simulink model "gm_sampleModel1449_sub"  (R2023a)
settings: Solver=VariableStepAuto  StartTime=0.0  StopTime=10.0  RelTol=1e-3
libraries: hdlsllib x1, simulink x1
settings Model: Creator=user1  LastModifiedBy=user1
settings OptimizationCC: BlockReduction=off  ConditionallyExecuteInputs=off
settings DebuggingCC: InheritedTsInSrcMsg=none

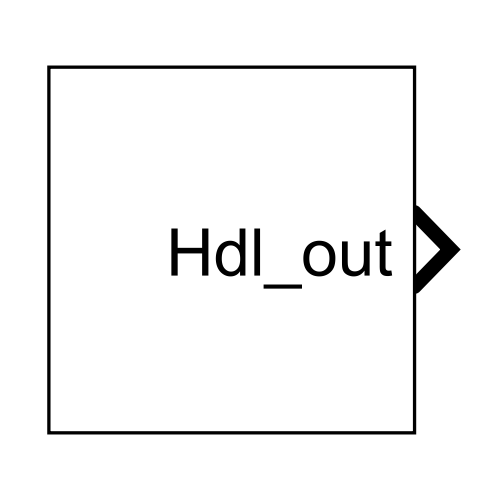
[thumbnail: Simulink's stored preview of the top-level diagram]
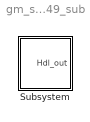
== system gm_sampleModel1449_sub ==
  Subsystem : Subsystem

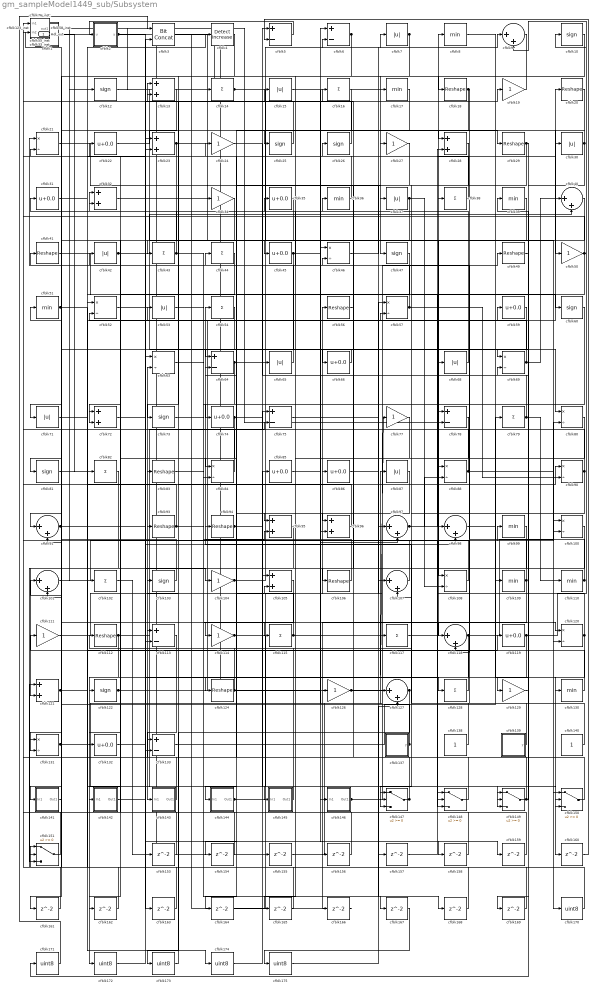
== system gm_sampleModel1449_sub/Subsystem ==
  cfblk1 : Subsystem  mask(Detect Rise Positive){vinit=double(0), InputProcessing=Elements as channels (sample based), OutDataTypeStr=uint8}
      mask prompts: vinit "Simulink:masks:InitialCondition_MP"; InputProcessing "Simulink:masks:InputProcessing_MP"; OutDataTypeStr "Simulink:masks:OutputDataType_MP"
      mask help: Simulink:masks:DetectRisePositive_MD
      mask init:
      | InputProcessing = 'Elements as channels (sample based)';
      | OutDataTypeStr = 'uint8';
      | vinit = double(0);
      mask TypeOptions InputProcessing: Simulink:masks:ColumnsAsChannelsFrameBased | Simulink:masks:ElementsAsChannelsSampleBased
      mask TypeOptions OutDataTypeStr: Simulink:masks:uint8 | Simulink:masks:boolean
      mask Display: fprintf('U > 0\n&  NOT\nU/z > 0')
  cfblk{10,12,25..26,47,60,73,81,103,122} (10 alike) : Signum
  cfblk{21,46,52,57,63,69,80,84,88,90,100,108,120,131} (14 alike) : Product  Inputs=*/  OutDataTypeStr=uint8  RndMeth=Zero  SaturateOnIntegerOverflow=on
  cfblk{9,40,91,97..98,101,107,118,127} (9 alike) : Sum  Inputs=|++  OutDataTypeStr=uint8
  cfblk{14,16,38,43..44,54,79,82,102,115,117,128} (12 alike) : Sum  Inputs=+  OutDataTypeStr=uint8
  cfblk{19,24,27,34,50,77,104,111,114,126,129} (11 alike) : Gain  OutDataTypeStr=uint8
  cfblk{13,23,28,32,72,95..96,105,121} (9 alike) : Sum  OutDataTypeStr=uint8
  cfblk{18,20,29,41,49,56,83,93..94,106,112,124} (12 alike) : Reshape
  cfblk{8,17,36,39,51,99,109..110,130} (9 alike) : MinMax  OutDataTypeStr=uint8
  cfblk{5..6,64,75,78,113,133} (7 alike) : Sum  Inputs=+-  OutDataTypeStr=uint8
  cfblk116_inst : Subsystem
  cfblk{22,31,35,45,59,66,74,85..86,119,132} (11 alike) : Bias  Bias=0.0  SaturateOnIntegerOverflow=off
  cfblk123_inst : Subsystem
  cfblk137 : Subsystem  mask(Counter Limited){uplimit=double(7), tsamp=double(-1)}
      mask prompts: uplimit "Simulink:masks:UpperLimit_MP"; tsamp "Simulink:masks:SampleTime_MP"
      mask help: Simulink:masks:CounterLimited_MD
      mask init:
      | nbits = double(8);
      | tsamp = double(-1);
      | uplimit = double(7);
  cfblk138 : Constant  OutDataTypeStr=uint8  SampleTime=-1
  cfblk139 : Subsystem  mask(Counter Free-Running){NumBits=double(16), tsamp=double(-1)}
      mask prompts: NumBits "Simulink:masks:NumberOfBits_MP"; tsamp "Simulink:masks:SampleTime_MP"
      mask help: Simulink:masks:CounterFreeRunning_MD
  cfblk140 : Constant  OutDataTypeStr=uint8  SampleTime=-1
  cfblk141 : Subsystem
  cfblk142 : Subsystem
  cfblk143 : Subsystem
  cfblk144 : Subsystem
  cfblk145 : Subsystem
  cfblk146 : Subsystem
  cfblk{147..151} (5 alike) : Switch  OutDataTypeStr=uint8  SaturateOnIntegerOverflow=off  InputSameDT=off
  cfblk{7,15,30,37,42,53,65,68,71,87} (10 alike) : Abs  OutDataTypeStr=uint8  SaturateOnIntegerOverflow=off
  cfblk{153..169} (17 alike) : Delay  SampleTime=1
  cfblk{170..175} (6 alike) : DataTypeConversion  OutDataTypeStr=uint8  SaturateOnIntegerOverflow=off  RndMeth=Floor
  cfblk2 : Subsystem  mask(Compare To Constant){relop=<=, const=double(3), OutDataTypeStr=uint8, ZeroCross=on}
      mask prompts: relop "Simulink:masks:Operator_MP"; const "Simulink:masks:ConstantValue_MP"; OutDataTypeStr "Simulink:masks:OutputDataType_MP"; ZeroCross "Simulink:masks:EnableZerocrossingDetection_MP"
      mask help: Simulink:masks:CompareToConstant_MD
      mask init:
      | OutDataTypeStr = 'uint8';
      | ZeroCross = 'on';
      | blkName = 'sampleModel1449_sub/Subsystem/cfblk2';
      | const = double(3);
      | const_str = '3.0';
      | const_val = double(3);
      | relop = '<=';
      | setValue = 'fixdt(0, 8)';
      | str = '<= 3';
      mask TypeOptions relop: == | ~= | < | <= | >= | >
      mask TypeOptions OutDataTypeStr: Simulink:masks:uint8 | Simulink:masks:boolean
      mask Callback ZeroCross: sl('zeroCrossEnable', gcbh);
      mask Display: disp(str)
  cfblk3 : hdlsllib/Logic and Bit Operations/Bit Concat  numInputs=2
  cfblk33_inst : Subsystem
  cfblk4 : simulink/Logic and Bit Operations/Detect Increase  vinit=0.0  OutDataTypeStr=uint8
      settings: LibrarySourceBlock=|
      | hdlsllib/Logic and Bit
      | Operations/Detect
      | Increase
  cfblk55_inst : Subsystem
  cfblk58_inst : Subsystem
  cfblk76_inst : Subsystem
  Hdl_out : Outport  OutDataTypeStr=uint8  SampleTime=1
  wires:
  cfblk1/1(Y) -> cfblk82/1
  cfblk10/1 -> cfblk47/1
  cfblk100/1 -> cfblk121/2
  cfblk101/1 -> cfblk99/1
  cfblk102/1 -> cfblk153/1
  cfblk103/1 -> cfblk55_inst/2(in2)
  cfblk104/1 -> cfblk6/2, cfblk90/1
  cfblk105/1 -> cfblk131/2
  cfblk106/1 -> cfblk54/1
  cfblk107/1 -> cfblk123_inst/2(in2)
  cfblk108/1 -> cfblk63/2
  cfblk109/1 -> cfblk41/1, cfblk166/1
  cfblk110/1 -> cfblk46/2, cfblk46/1, cfblk39/1
  cfblk111/1 -> cfblk105/2
  cfblk112/1 -> cfblk75/2, cfblk75/1, cfblk172/1, cfblk147/3
  cfblk113/1 -> cfblk143/1(In1)
  cfblk114/1 -> cfblk56/1, cfblk149/3
  cfblk115/1 -> cfblk49/1, cfblk44/1
  cfblk116_inst/1(out1) -> cfblk17/1
  cfblk117/1 -> cfblk8/1
  cfblk118/1 -> cfblk122/1, cfblk80/2
  cfblk119/1 -> cfblk9/2, cfblk126/1
  cfblk12/1 -> cfblk45/1
  cfblk120/1 -> cfblk160/1, cfblk38/1
  cfblk121/1 -> cfblk86/1, cfblk59/1, cfblk119/1
  cfblk122/1 -> cfblk23/2, cfblk20/1
  cfblk123_inst/1(out1) -> cfblk102/1
  cfblk124/1 -> cfblk97/2, cfblk83/1
  cfblk126/1 -> cfblk77/1, cfblk16/1
  cfblk127/1 -> cfblk173/1, Hdl_out/1
  cfblk128/1 -> cfblk52/2
  cfblk129/1 -> cfblk171/1
  cfblk13/1 -> cfblk71/1
  cfblk130/1 -> cfblk111/1
  cfblk131/1 -> cfblk87/1, cfblk150/3
  cfblk132/1 -> cfblk163/1
  cfblk133/1 -> cfblk79/1
  cfblk137/1(y) -> cfblk6/1, cfblk21/2
  cfblk138/1 -> cfblk112/1
  cfblk139/1(y) -> cfblk94/1
  cfblk14/1 -> cfblk108/1, cfblk100/2
  cfblk140/1 -> cfblk98/1
  cfblk141/1(Out1) -> cfblk51/1
  cfblk142/1(Out1) -> cfblk158/1
  cfblk143/1(Out1) -> cfblk33_inst/1(in1)
  cfblk144/1(Out1) -> cfblk85/1, cfblk28/2
  cfblk145/1(Out1) -> cfblk105/1
  cfblk146/1(Out1) -> cfblk68/1, cfblk149/2
  cfblk147/1 -> cfblk93/1, cfblk113/1
  cfblk148/1 -> cfblk64/2
  cfblk149/1 -> cfblk69/2, cfblk63/1
  cfblk15/1 -> cfblk159/1
  cfblk150/1 -> cfblk36/1
  cfblk151/1 -> cfblk58_inst/1(in1)
  cfblk153/1 -> cfblk58_inst/2(in2)
  cfblk154/1 -> cfblk32/1
  cfblk155/1 -> cfblk88/1
  cfblk156/1 -> cfblk13/1
  cfblk157/1 -> cfblk100/1
  cfblk158/1 -> cfblk101/1
  cfblk159/1 -> cfblk131/1
  cfblk16/1 -> cfblk124/1
  cfblk160/1 -> cfblk5/2
  cfblk161/1 -> cfblk55_inst/1(in1)
  cfblk162/1 -> cfblk151/1
  cfblk163/1 -> cfblk91/2
  cfblk164/1 -> cfblk57/1
  cfblk165/1 -> cfblk133/1
  cfblk166/1 -> cfblk1/1(U)
  cfblk167/1 -> cfblk175/1
  cfblk168/1 -> cfblk121/1
  cfblk169/1 -> cfblk151/2
  cfblk17/1 -> cfblk25/1
  cfblk170/1 -> cfblk52/1
  cfblk171/1 -> cfblk3/1
  cfblk172/1 -> cfblk3/2
  cfblk173/1 -> cfblk103/1
  cfblk174/1 -> cfblk127/1
  cfblk175/1 -> cfblk127/2
  cfblk18/1 -> cfblk118/2, cfblk27/1
  cfblk19/1 -> cfblk18/1
  cfblk2/1(y) -> cfblk104/1, cfblk128/1
  cfblk20/1 -> cfblk50/1
  cfblk21/1 -> cfblk157/1
  cfblk22/1 -> cfblk29/1
  cfblk23/1 -> cfblk37/1, cfblk162/1
  cfblk24/1 -> cfblk65/1
  cfblk25/1 -> cfblk15/1
  cfblk26/1 -> cfblk76_inst/2(in2)
  cfblk27/1 -> cfblk96/1
  cfblk28/1 -> cfblk74/1
  cfblk29/1 -> cfblk147/2, cfblk129/1
  cfblk3/1 -> cfblk170/1
  cfblk30/1 -> cfblk28/1, cfblk69/1
  cfblk31/1 -> cfblk4/1
  cfblk32/1 -> cfblk97/1
  cfblk33_inst/1(out1) -> cfblk78/2
  cfblk34/1 -> cfblk132/1
  cfblk35/1 -> cfblk141/1(In1)
  cfblk36/1 -> cfblk76_inst/1(in1)
  cfblk37/1 -> cfblk72/2, cfblk108/2
  cfblk38/1 -> cfblk116_inst/1(in1)
  cfblk39/1 -> cfblk164/1
  cfblk4/1 -> cfblk73/1
  cfblk40/1 -> cfblk66/1
  cfblk41/1 -> cfblk148/1
  cfblk42/1 -> cfblk40/2, cfblk80/1
  cfblk43/1 -> cfblk31/1, cfblk167/1
  cfblk44/1 -> cfblk72/1
  cfblk45/1 -> cfblk7/1, cfblk113/2
  cfblk46/1 -> cfblk9/1
  cfblk47/1 -> cfblk114/1
  cfblk49/1 -> cfblk169/1
  cfblk5/1 -> cfblk2/1(u)
  cfblk50/1 -> cfblk147/1, cfblk116_inst/2(in2), cfblk10/1
  cfblk51/1 -> cfblk60/1, cfblk174/1
  cfblk52/1 -> cfblk107/1
  cfblk53/1 -> cfblk57/2
  cfblk54/1 -> cfblk91/1
  cfblk55_inst/1(out1) -> cfblk12/1
  cfblk56/1 -> cfblk26/1
  cfblk57/1 -> cfblk35/1, cfblk90/2
  cfblk58_inst/1(out1) -> cfblk14/1
  cfblk59/1 -> cfblk106/1
  cfblk6/1 -> cfblk81/1, cfblk161/1
  cfblk60/1 -> cfblk84/1
  cfblk63/1 -> cfblk156/1
  cfblk64/1 -> cfblk150/2, cfblk84/2, cfblk24/1
  cfblk65/1 -> cfblk21/1
  cfblk66/1 -> cfblk64/1
  cfblk68/1 -> cfblk22/1
  cfblk69/1 -> cfblk42/1, cfblk40/1
  cfblk7/1 -> cfblk101/2, cfblk43/1
  cfblk71/1 -> cfblk145/1(In1)
  cfblk72/1 -> cfblk34/1
  cfblk73/1 -> cfblk117/1
  cfblk74/1 -> cfblk120/1, cfblk142/1(In1)
  cfblk75/1 -> cfblk118/1
  cfblk76_inst/1(out1) -> cfblk155/1
  cfblk77/1 -> cfblk96/2
  cfblk78/1 -> cfblk95/1
  cfblk79/1 -> cfblk5/1, cfblk110/1
  cfblk8/1 -> cfblk109/1
  cfblk80/1 -> cfblk148/2
  cfblk81/1 -> cfblk23/1
  cfblk82/1 -> cfblk151/3
  cfblk83/1 -> cfblk115/1
  cfblk84/1 -> cfblk123_inst/1(in1)
  cfblk85/1 -> cfblk146/1(In1)
  cfblk86/1 -> cfblk168/1
  cfblk87/1 -> cfblk144/1(In1)
  cfblk88/1 -> cfblk78/1, cfblk150/1
  cfblk9/1 -> cfblk165/1
  cfblk90/1 -> cfblk32/2, cfblk107/2
  cfblk91/1 -> cfblk98/2, cfblk19/1
  cfblk93/1 -> cfblk95/2, cfblk53/1, cfblk33_inst/2(in2)
  cfblk94/1 -> cfblk148/3, cfblk120/2
  cfblk95/1 -> cfblk154/1
  cfblk96/1 -> cfblk13/2
  cfblk97/1 -> cfblk30/1, cfblk149/1, cfblk88/2
  cfblk98/1 -> cfblk130/1
  cfblk99/1 -> cfblk133/2

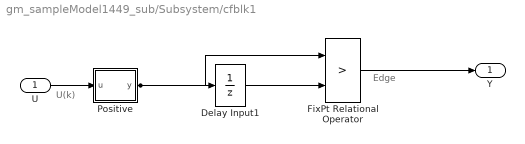
== system gm_sampleModel1449_sub/Subsystem/cfblk1 ==
  note: U(k)
  note: Edge
  U : Inport  OutDataTypeStr=uint8  SampleTime=1
  Delay Input1 : UnitDelay  Description=Store in Global RAM  DisableCoverage=on  InitialCondition=vinit  SampleTime=-1  HasFrameUpgradeWarning=on
  FixPt Relational Operator : RelationalOperator  Operator=>  OutDataTypeStr=fixdt(0, 8)  ZeroCross=off  InputSameDT=off
  Positive : Subsystem  mask(Compare To Zero){relop=>, OutDataTypeStr=boolean, ZeroCross=off}
      mask prompts: relop "Simulink:masks:Operator_MP"; OutDataTypeStr "Simulink:masks:OutputDataType_MP"; ZeroCross "Simulink:masks:EnableZerocrossingDetection_MP"
      mask help: Simulink:masks:CompareToZero_MD
      mask init:
      | OutDataTypeStr = 'boolean';
      | ZeroCross = 'off';
      | blkName = 'sampleModel1449_sub/Subsystem/cfblk1/Positive';
      | relop = '>';
      | setValue = 'boolean';
      mask TypeOptions relop: == | ~= | < | <= | >= | >
      mask TypeOptions OutDataTypeStr: Simulink:masks:uint8 | Simulink:masks:boolean
      mask Callback ZeroCross: sl('zeroCrossEnable', gcbh);
      mask Display: disp([relop,' 0'])
  Y : Outport  SampleTime=1
  wires:
  U/1 -> Positive/1(u)
  Delay Input1/1 -> FixPt Relational Operator/2
  FixPt Relational Operator/1 -> Y/1
  Positive/1(y) -> FixPt Relational Operator/1, Delay Input1/1

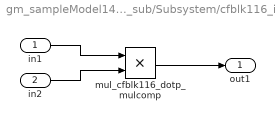
== system gm_sampleModel1449_sub/Subsystem/cfblk116_inst ==
  in1 : Inport  OutDataTypeStr=uint8  SampleTime=1
  in2 : Inport  Port=2  OutDataTypeStr=uint8  SampleTime=1
  mul_cfblk116_dotp_mulcomp : Product  Inputs=**  OutDataTypeStr=uint8  SampleTime=1
  out1 : Outport  OutDataTypeStr=uint8  SampleTime=1
  wires:
  in1/1 -> mul_cfblk116_dotp_mulcomp/1
  in2/1 -> mul_cfblk116_dotp_mulcomp/2
  mul_cfblk116_dotp_mulcomp/1 -> out1/1

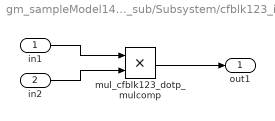
== system gm_sampleModel1449_sub/Subsystem/cfblk123_inst ==
  in1 : Inport  OutDataTypeStr=uint8  SampleTime=1
  in2 : Inport  Port=2  OutDataTypeStr=uint8  SampleTime=1
  mul_cfblk123_dotp_mulcomp : Product  Inputs=**  OutDataTypeStr=uint8  SampleTime=1
  out1 : Outport  OutDataTypeStr=uint8  SampleTime=1
  wires:
  in1/1 -> mul_cfblk123_dotp_mulcomp/1
  in2/1 -> mul_cfblk123_dotp_mulcomp/2
  mul_cfblk123_dotp_mulcomp/1 -> out1/1

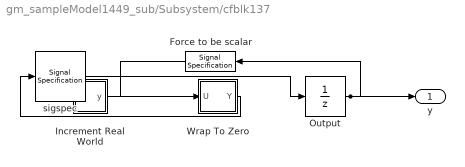
== system gm_sampleModel1449_sub/Subsystem/cfblk137 ==
  Force to be scalar : SignalSpecification  DisableCoverage=on  Dimensions=1
  Increment Real World : Subsystem  mask(Real World Value Increment){}
      mask help: Simulink:masks:RealWorldValueIncrement_MD
      mask Display: disp('V++')
  Output : UnitDelay  InitialCondition=0.0  SampleTime=tsamp  HasFrameUpgradeWarning=on
  Wrap To Zero : Subsystem  mask(Wrap To Zero){Threshold=double(7)}
      mask prompts: Threshold "Simulink:masks:Threshold_MP"
      mask help: Simulink:masks:WrapToZero_MD
  sigspec : SignalSpecification  OutDataTypeStr=uint8  Dimensions=1
  y : Outport  SampleTime=1
  wires:
  Force to be scalar/1 -> Increment Real World/1(u)
  Increment Real World/1(y) -> Wrap To Zero/1(U)
  Output/1 -> Force to be scalar/1, y/1
  Wrap To Zero/1(Y) -> sigspec/1
  sigspec/1 -> Output/1

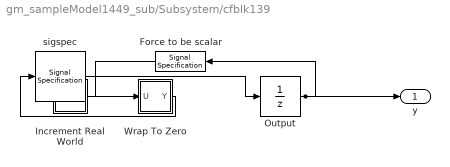
== system gm_sampleModel1449_sub/Subsystem/cfblk139 ==
  Force to be scalar : SignalSpecification  DisableCoverage=on  Dimensions=1
  Increment Real World : Subsystem  mask(Real World Value Increment){}
      mask help: Simulink:masks:RealWorldValueIncrement_MD
      mask Display: disp('V++')
  Output : UnitDelay  InitialCondition=0.0  SampleTime=tsamp  HasFrameUpgradeWarning=on
  Wrap To Zero : Subsystem  mask(Wrap To Zero){Threshold=double(65535)}
      mask prompts: Threshold "Simulink:masks:Threshold_MP"
      mask help: Simulink:masks:WrapToZero_MD
  sigspec : SignalSpecification  OutDataTypeStr=uint16  Dimensions=1
  y : Outport  SampleTime=1
  wires:
  Force to be scalar/1 -> Increment Real World/1(u)
  Increment Real World/1(y) -> Wrap To Zero/1(U)
  Output/1 -> Force to be scalar/1, y/1
  Wrap To Zero/1(Y) -> sigspec/1
  sigspec/1 -> Output/1

== system gm_sampleModel1449_sub/Subsystem/cfblk141 ==
  In1 : Inport  OutDataTypeStr=uint8  PortDimensions=1  SampleTime=1
  Out1 : Outport  SampleTime=1
  wires:
  In1/1 -> Out1/1

== system gm_sampleModel1449_sub/Subsystem/cfblk142 ==
  In1 : Inport  OutDataTypeStr=uint8  PortDimensions=1  SampleTime=1
  Out1 : Outport  SampleTime=1
  wires:
  In1/1 -> Out1/1

== system gm_sampleModel1449_sub/Subsystem/cfblk143 ==
  In1 : Inport  OutDataTypeStr=uint8  PortDimensions=1  SampleTime=1
  Out1 : Outport  SampleTime=1
  wires:
  In1/1 -> Out1/1

== system gm_sampleModel1449_sub/Subsystem/cfblk144 ==
  In1 : Inport  OutDataTypeStr=uint8  PortDimensions=1  SampleTime=1
  Out1 : Outport  SampleTime=1
  wires:
  In1/1 -> Out1/1

== system gm_sampleModel1449_sub/Subsystem/cfblk145 ==
  In1 : Inport  OutDataTypeStr=uint8  PortDimensions=1  SampleTime=1
  Out1 : Outport  SampleTime=1
  wires:
  In1/1 -> Out1/1

== system gm_sampleModel1449_sub/Subsystem/cfblk146 ==
  In1 : Inport  OutDataTypeStr=uint8  PortDimensions=1  SampleTime=1
  Out1 : Outport  SampleTime=1
  wires:
  In1/1 -> Out1/1

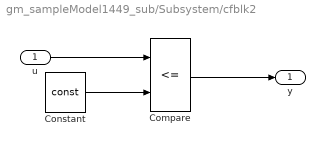
== system gm_sampleModel1449_sub/Subsystem/cfblk2 ==
  u : Inport  OutDataTypeStr=uint8  SampleTime=1
  Compare : RelationalOperator  Operator=<=  OutDataTypeStr=fixdt(0, 8)
  Constant : Constant  DisableCoverage=on  Value=const  OutDataTypeStr=Inherit: Inherit via back propagation  SampleTime=-1
  y : Outport  SampleTime=1
  wires:
  u/1 -> Compare/1
  Compare/1 -> y/1
  Constant/1 -> Compare/2

== system gm_sampleModel1449_sub/Subsystem/cfblk33_inst ==
  in1 : Inport  OutDataTypeStr=uint8  SampleTime=1
  in2 : Inport  Port=2  OutDataTypeStr=uint8  SampleTime=1
  mul_cfblk33_dotp_mulcomp : Product  Inputs=**  OutDataTypeStr=uint8  SampleTime=1
  out1 : Outport  OutDataTypeStr=uint8  SampleTime=1
  wires:
  in1/1 -> mul_cfblk33_dotp_mulcomp/1
  in2/1 -> mul_cfblk33_dotp_mulcomp/2
  mul_cfblk33_dotp_mulcomp/1 -> out1/1

== system gm_sampleModel1449_sub/Subsystem/cfblk55_inst ==
  in1 : Inport  OutDataTypeStr=uint8  SampleTime=1
  in2 : Inport  Port=2  OutDataTypeStr=uint8  SampleTime=1
  mul_cfblk55_dotp_mulcomp : Product  Inputs=**  OutDataTypeStr=uint8  SampleTime=1
  out1 : Outport  OutDataTypeStr=uint8  SampleTime=1
  wires:
  in1/1 -> mul_cfblk55_dotp_mulcomp/1
  in2/1 -> mul_cfblk55_dotp_mulcomp/2
  mul_cfblk55_dotp_mulcomp/1 -> out1/1

== system gm_sampleModel1449_sub/Subsystem/cfblk58_inst ==
  in1 : Inport  OutDataTypeStr=uint8  SampleTime=1
  in2 : Inport  Port=2  OutDataTypeStr=uint8  SampleTime=1
  mul_cfblk58_dotp_mulcomp : Product  Inputs=**  OutDataTypeStr=uint8  SampleTime=1
  out1 : Outport  OutDataTypeStr=uint8  SampleTime=1
  wires:
  in1/1 -> mul_cfblk58_dotp_mulcomp/1
  in2/1 -> mul_cfblk58_dotp_mulcomp/2
  mul_cfblk58_dotp_mulcomp/1 -> out1/1

== system gm_sampleModel1449_sub/Subsystem/cfblk76_inst ==
  in1 : Inport  OutDataTypeStr=uint8  SampleTime=1
  in2 : Inport  Port=2  OutDataTypeStr=uint8  SampleTime=1
  mul_cfblk76_dotp_mulcomp : Product  Inputs=**  OutDataTypeStr=uint8  SampleTime=1
  out1 : Outport  OutDataTypeStr=uint8  SampleTime=1
  wires:
  in1/1 -> mul_cfblk76_dotp_mulcomp/1
  in2/1 -> mul_cfblk76_dotp_mulcomp/2
  mul_cfblk76_dotp_mulcomp/1 -> out1/1

== system gm_sampleModel1449_sub/Subsystem/cfblk1/Positive ==
  u : Inport  OutDataTypeStr=uint8  SampleTime=1
  Compare : RelationalOperator  Operator=>  OutDataTypeStr=boolean  ZeroCross=off
  Constant : Constant  DisableCoverage=on  Value=0  OutDataTypeStr=Inherit: Inherit via back propagation  SampleTime=-1  PreserveConstantTs=on
  y : Outport  SampleTime=1
  wires:
  u/1 -> Compare/1
  Compare/1 -> y/1
  Constant/1 -> Compare/2

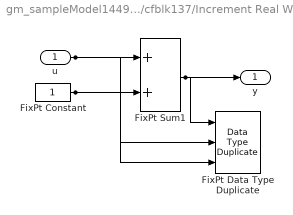
== system gm_sampleModel1449_sub/Subsystem/cfblk137/Increment Real World ==
  u : Inport  OutDataTypeStr=uint8  SampleTime=1
  FixPt Constant : Constant  DisableCoverage=on  OutDataTypeStr=Inherit: Inherit via back propagation  SampleTime=-1
  FixPt Data Type Duplicate : DataTypeDuplicate  DisableCoverage=on  NumInputPorts=3
  FixPt Sum1 : Sum  InputSameDT=on  OutDataTypeStr=Inherit: Inherit via back propagation  LockScale=on
  y : Outport  SampleTime=1
  wires:
  u/1 -> FixPt Sum1/1, FixPt Data Type Duplicate/2
  FixPt Constant/1 -> FixPt Sum1/2, FixPt Data Type Duplicate/3
  FixPt Sum1/1 -> FixPt Data Type Duplicate/1, y/1

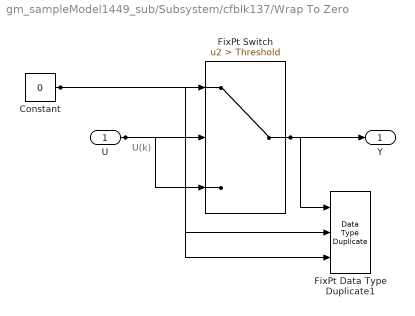
== system gm_sampleModel1449_sub/Subsystem/cfblk137/Wrap To Zero ==
  note: U(k)
  U : Inport  OutDataTypeStr=uint8  SampleTime=1
  Constant : Constant  DisableCoverage=on  Value=0  OutDataTypeStr=Inherit: Inherit via back propagation  SampleTime=-1
  FixPt Data Type Duplicate1 : DataTypeDuplicate  DisableCoverage=on  NumInputPorts=3
  FixPt Switch : Switch  Criteria=u2 > Threshold  Threshold=Threshold  OutDataTypeStr=Inherit: Inherit via back propagation  ZeroCross=off  SaturateOnIntegerOverflow=off  InputSameDT=off
  Y : Outport  SampleTime=1
  wires:
  U/1 -> FixPt Switch/3, FixPt Switch/2, FixPt Data Type Duplicate1/2
  Constant/1 -> FixPt Switch/1, FixPt Data Type Duplicate1/3
  FixPt Switch/1 -> FixPt Data Type Duplicate1/1, Y/1

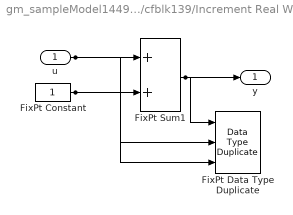
== system gm_sampleModel1449_sub/Subsystem/cfblk139/Increment Real World ==
  u : Inport  OutDataTypeStr=uint16  SampleTime=1
  FixPt Constant : Constant  DisableCoverage=on  OutDataTypeStr=Inherit: Inherit via back propagation  SampleTime=-1
  FixPt Data Type Duplicate : DataTypeDuplicate  DisableCoverage=on  NumInputPorts=3
  FixPt Sum1 : Sum  InputSameDT=on  OutDataTypeStr=Inherit: Inherit via back propagation  LockScale=on
  y : Outport  SampleTime=1
  wires:
  u/1 -> FixPt Sum1/1, FixPt Data Type Duplicate/2
  FixPt Constant/1 -> FixPt Sum1/2, FixPt Data Type Duplicate/3
  FixPt Sum1/1 -> FixPt Data Type Duplicate/1, y/1

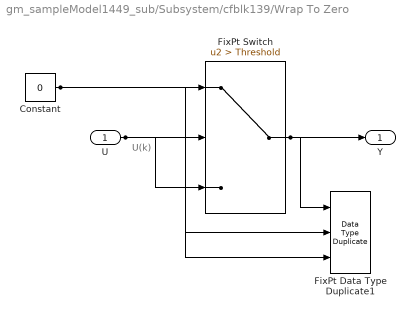
== system gm_sampleModel1449_sub/Subsystem/cfblk139/Wrap To Zero ==
  note: U(k)
  U : Inport  OutDataTypeStr=uint16  SampleTime=1
  Constant : Constant  DisableCoverage=on  Value=0  OutDataTypeStr=Inherit: Inherit via back propagation  SampleTime=-1
  FixPt Data Type Duplicate1 : DataTypeDuplicate  DisableCoverage=on  NumInputPorts=3
  FixPt Switch : Switch  Criteria=u2 > Threshold  Threshold=Threshold  OutDataTypeStr=Inherit: Inherit via back propagation  ZeroCross=off  SaturateOnIntegerOverflow=off  InputSameDT=off
  Y : Outport  SampleTime=1
  wires:
  U/1 -> FixPt Switch/3, FixPt Switch/2, FixPt Data Type Duplicate1/2
  Constant/1 -> FixPt Switch/1, FixPt Data Type Duplicate1/3
  FixPt Switch/1 -> FixPt Data Type Duplicate1/1, Y/1
